simulink model "es728_3simulink"  (R2024b)
settings: Solver=VariableStepAuto  StartTime=0.0  StopTime=10.0  RelTol=1e-3
values from neighbouring files (symbols this model uses):
  A = [0,   0,   1,    0 ... (first row only)    [es728_1.m]    (also in es728_2.m; es728_3.m)
  B = [ 0; 0; 1/mc;  1/(L*mc)]    [es728_1.m]    (also in es728_2.m; es728_3.m)
  D = 0    [es728_1.m]    (also in es728_2.m; es728_3.m)
  K = acker(A,B,des_poles)    [es728_3.m]
settings Model: Creator=njsne  LastModifiedBy=njsne

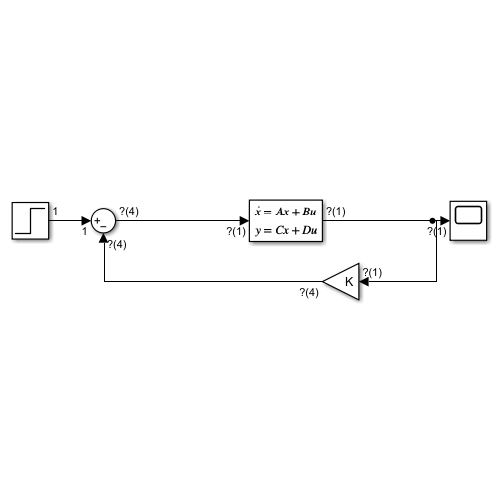
[thumbnail: Simulink's stored preview of the top-level diagram]
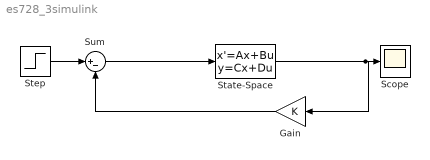
== system es728_3simulink ==
  Gain : Gain  Gain=K
  Scope : Scope
  State-Space : StateSpace  A=A  B=B  C=[1 0 0 0]  D=D  InitialCondition=[0.1;0.174533;0;0]
  Step : Step  Time=0  After=0.0  SampleTime=0
  Sum : Sum  Inputs=|+-
  wires:
  Step/1 -> Sum/1
  State-Space/1 -> Gain/1, Scope/1
  Gain/1 -> Sum/2
  Sum/1 -> State-Space/1
